simulink model "a340_simulink"  (R2018b)
settings: Solver=VariableStepAuto  StartTime=0.0  StopTime=100  RelTol=1e-3  EnableMultiTasking=on
values from neighbouring files (symbols this model uses):
  A = [sys_yaw_dynamics, sys_roll2yaw_couple ... (first row only)    [main.m]
  B = [input_yaw_dynamics, input_roll2yaw_couple ... (first row only)    [main.m]
  C = [output_yaw, [0 0] ... (first row only)    [main.m]
  K_lqr = lqr(A,B,Q,R)    [main.m]
  K_lqr_dis1 = lqrd(A,B,Q,R, 0.2)    [main.m]
  K_lqr_dis2 = lqrd(A,B,Q,R, 1)    [main.m]
  K_lqr_dis3 = lqrd(A,B,Q,R, 2)    [main.m]
  Kr_lqr = -(E*((A-B*K_lqr)^-1)*B)^-1    [main.m]
  Kr_lqr_dis1 = -(E*((A-B*K_lqr_dis1)^-1)*B)^-1    [main.m]
  Kr_lqr_dis2 = -(E*((A-B*K_lqr_dis2)^-1)*B)^-1    [main.m]
  Kr_lqr_dis3 = -(E*((A-B*K_lqr_dis3)^-1)*B)^-1    [main.m]
libraries: simulink x1
settings Model: Creator=user  LastModifiedBy=john
settings OptimizationCC: LifeSpan=inf
settings DebuggingCC: SFUnexpectedBacktrackingDiag=warning  SFNoUnconditionalDefaultTransitionDiag=warning
settings SFSimCC: SimUseLocalCustomCode=off
settings RTWCC: RTWUseLocalCustomCode=off
settings CodeAppCC: StateflowObjectComments=on
settings GRTTargetCC: TargetLangStandard=C89/C90 (ANSI)  GeneratePreprocessorConditionals=Disable all
settings ConfigComp: CovMetricSettings=dw  CovHtmlReporting=on  CovSaveCumulativeToWorkspaceVar=on  CovSaveSingleToWorkspaceVar=on  CovExternalEMLEnable=off

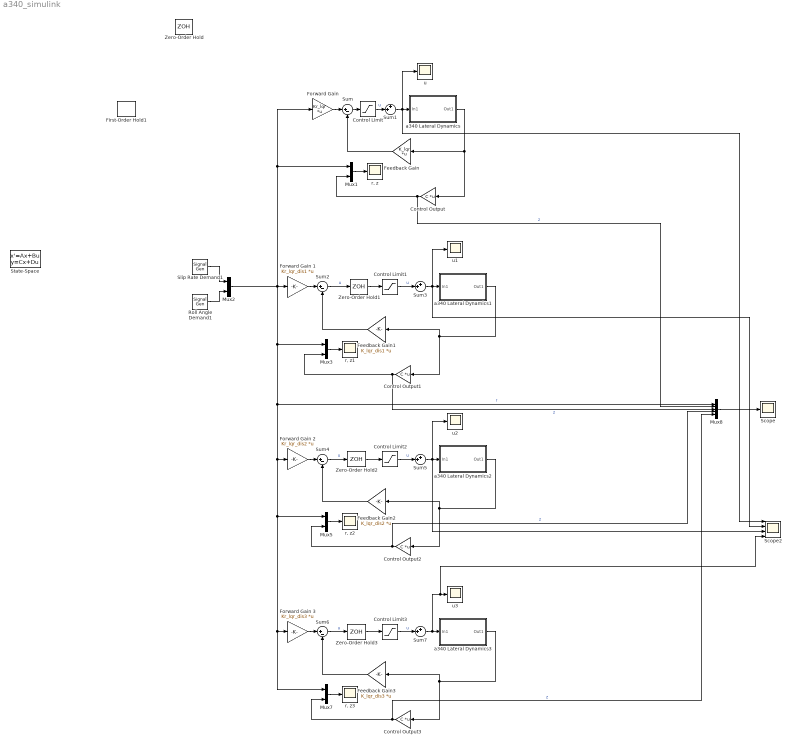
== system a340_simulink ==
  Control Limit{,1..3} (4 alike) : Saturate  UpperLimit=0.2  LowerLimit=-0.2
  Control Output{,1..3} (4 alike) : Gain  Gain=C  Multiplication=Matrix(K*u)
  Feedback Gain : Gain  Gain=K_lqr  Multiplication=Matrix(K*u)
  Feedback Gain1 : Gain  Gain=K_lqr_dis1  Multiplication=Matrix(K*u)
  Feedback Gain2 : Gain  Gain=K_lqr_dis2  Multiplication=Matrix(K*u)
  Feedback Gain3 : Gain  Gain=K_lqr_dis3  Multiplication=Matrix(K*u)
  First-Order Hold1 : simulink/Discrete/First-Order Hold  DisableCoverage=on  Ts=0.1
      settings: SourceProductName=Simulink  SourceProductBaseCode=SL
  "Forward Gain " : Gain  Gain=Kr_lqr  Multiplication=Matrix(K*u)
  Forward Gain 1 : Gain  Gain=Kr_lqr_dis1  Multiplication=Matrix(K*u)
  Forward Gain 2 : Gain  Gain=Kr_lqr_dis2  Multiplication=Matrix(K*u)
  Forward Gain 3 : Gain  Gain=Kr_lqr_dis3  Multiplication=Matrix(K*u)
  Mux{1..3,5,7} (5 alike) : Mux  Inputs=2
  Mux8 : Mux  Inputs=5
  Roll Angle Demand1 : SignalGenerator  WaveForm=square  Amplitude=0.1  Frequency=0.1
  Scope : Scope
  Scope2 : Scope  NumInputPorts=4
  Slip Rate Demand1 : SignalGenerator  Amplitude=0.5  Frequency=0.05
  State-Space : StateSpace  InitialCondition=0  ContinuousStateAttributes='position'
  Sum{,2,4,6} (4 alike) : Sum  Inputs=|+-
  Sum{1,3,5,7} (4 alike) : Sum  Inputs=++|
  Zero-Order Hold : ZeroOrderHold  SampleTime=-1
  Zero-Order Hold1 : ZeroOrderHold  SampleTime=0.2
  Zero-Order Hold2 : ZeroOrderHold
  Zero-Order Hold3 : ZeroOrderHold  SampleTime=2
  a340 Lateral Dynamics : Subsystem
      mask Display: image('airbus-a340-blade-clean-sky-project.jpg');
  a340 Lateral Dynamics1 : Subsystem
      mask Display: image('airbus-a340-blade-clean-sky-project.jpg');
  a340 Lateral Dynamics2 : Subsystem
      mask Display: image('airbus-a340-blade-clean-sky-project.jpg');
  a340 Lateral Dynamics3 : Subsystem
      mask Display: image('airbus-a340-blade-clean-sky-project.jpg');
  r, z{,1..3} (4 alike) : Scope
  u{,1..3} (4 alike) : Scope
  wires:
  "Forward Gain "/1 -> Sum/1
  Sum/1 -> Control Limit/1
  a340 Lateral Dynamics/1(Out1) -> Control Output/1, Feedback Gain/1
  Mux1/1 -> "r, z"/1
  Control Output/1 -> Mux8/2, Mux1/2  "z"
  Feedback Gain/1 -> Sum/2
  Control Limit/1 -> Sum1/2  "u"
  Sum1/1 -> Scope2/1, u/1, a340 Lateral Dynamics/1(In1)
  Slip Rate Demand1/1 -> Mux2/1
  Roll Angle Demand1/1 -> Mux2/2
  Sum3/1 -> Scope2/2, u1/1, a340 Lateral Dynamics1/1(In1)
  Sum2/1 -> Zero-Order Hold1/1  "u"
  Feedback Gain1/1 -> Sum2/2
  Mux3/1 -> "r, z1"/1
  Forward Gain 1/1 -> Sum2/1
  Mux2/1 -> Mux7/1, Forward Gain 3/1, Mux5/1, Forward Gain 2/1, Mux8/1, Mux3/1, Mux1/1, "Forward Gain "/1, Forward Gain 1/1  "r"
  Control Limit1/1 -> Sum3/2  "u"
  a340 Lateral Dynamics1/1(Out1) -> Feedback Gain1/1, Control Output1/1
  Zero-Order Hold1/1 -> Control Limit1/1
  Zero-Order Hold2/1 -> Control Limit2/1
  Sum4/1 -> Zero-Order Hold2/1  "u"
  Control Limit2/1 -> Sum5/2  "u"
  Sum5/1 -> Scope2/3, u2/1, a340 Lateral Dynamics2/1(In1)
  Forward Gain 2/1 -> Sum4/1
  Control Output2/1 -> Mux8/4, Mux5/2  "z"
  a340 Lateral Dynamics2/1(Out1) -> Feedback Gain2/1, Control Output2/1
  Mux5/1 -> "r, z2"/1
  Feedback Gain2/1 -> Sum4/2
  Zero-Order Hold3/1 -> Control Limit3/1
  Sum6/1 -> Zero-Order Hold3/1  "u"
  Control Limit3/1 -> Sum7/2  "u"
  Sum7/1 -> Scope2/4, u3/1, a340 Lateral Dynamics3/1(In1)
  Forward Gain 3/1 -> Sum6/1
  Control Output3/1 -> Mux8/5, Mux7/2  "z"
  a340 Lateral Dynamics3/1(Out1) -> Feedback Gain3/1, Control Output3/1
  Mux7/1 -> "r, z3"/1
  Feedback Gain3/1 -> Sum6/2
  Mux8/1 -> Scope/1
  Control Output1/1 -> Mux8/3, Mux3/2  "z"

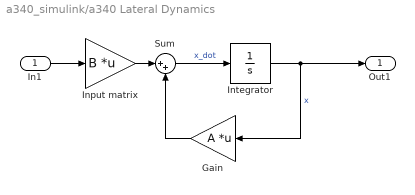
== system a340_simulink/a340 Lateral Dynamics ==
  In1 : Inport
  Gain : Gain  Gain=A  Multiplication=Matrix(K*u)
  Input matrix : Gain  Gain=B  Multiplication=Matrix(K*u) (u vector)
  Integrator : Integrator  InitialCondition=[-0.2 0.2 0.1 -0.1]
  Sum : Sum  Inputs=|++
  Out1 : Outport
  wires:
  In1/1 -> Input matrix/1
  Sum/1 -> Integrator/1  "x_dot"
  Integrator/1 -> Out1/1, Gain/1  "x"
  Input matrix/1 -> Sum/1
  Gain/1 -> Sum/2

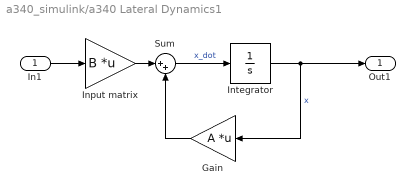
== system a340_simulink/a340 Lateral Dynamics1 ==
  In1 : Inport
  Gain : Gain  Gain=A  Multiplication=Matrix(K*u)
  Input matrix : Gain  Gain=B  Multiplication=Matrix(K*u) (u vector)
  Integrator : Integrator  InitialCondition=[-0.2 0.2 0.1 -0.1]
  Sum : Sum  Inputs=|++
  Out1 : Outport
  wires:
  In1/1 -> Input matrix/1
  Sum/1 -> Integrator/1  "x_dot"
  Integrator/1 -> Out1/1, Gain/1  "x"
  Input matrix/1 -> Sum/1
  Gain/1 -> Sum/2

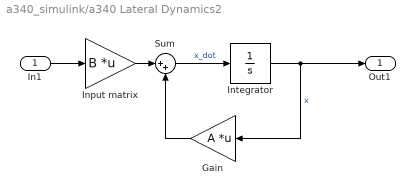
== system a340_simulink/a340 Lateral Dynamics2 ==
  In1 : Inport
  Gain : Gain  Gain=A  Multiplication=Matrix(K*u)
  Input matrix : Gain  Gain=B  Multiplication=Matrix(K*u) (u vector)
  Integrator : Integrator  InitialCondition=[-0.2 0.2 0.1 -0.1]
  Sum : Sum  Inputs=|++
  Out1 : Outport
  wires:
  In1/1 -> Input matrix/1
  Sum/1 -> Integrator/1  "x_dot"
  Integrator/1 -> Out1/1, Gain/1  "x"
  Input matrix/1 -> Sum/1
  Gain/1 -> Sum/2

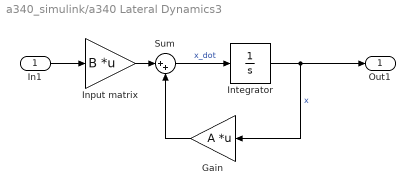
== system a340_simulink/a340 Lateral Dynamics3 ==
  In1 : Inport
  Gain : Gain  Gain=A  Multiplication=Matrix(K*u)
  Input matrix : Gain  Gain=B  Multiplication=Matrix(K*u) (u vector)
  Integrator : Integrator  InitialCondition=[-0.2 0.2 0.1 -0.1]
  Sum : Sum  Inputs=|++
  Out1 : Outport
  wires:
  In1/1 -> Input matrix/1
  Sum/1 -> Integrator/1  "x_dot"
  Integrator/1 -> Out1/1, Gain/1  "x"
  Input matrix/1 -> Sum/1
  Gain/1 -> Sum/2
